simulink model "body_assembly"  (R2023b)
settings: Solver=VariableStepAuto  StartTime=0.0  StopTime=10.0  RelTol=1e-3
model workspace: external: MATLAB File S:\sabik\projects\3-1 project\3d modelling\body assembly 6\matlab_simulation\body_assembly_DataFile.m (data not in the file)
undefined symbols (not defined in the file or in its folder): smiData, X, Y, Z
libraries: sm_lib x393, nesl_utility x25, slpidlib x12
(part 8 of 8)

== system body_assembly/rocko_model/femur_fl/Assembly_SERVO_1_RIGID/Assembly_SERVO_stp_1_RIGID/Assembly_servo_inside_stp_1_RIGID ==
  ReferenceFrame : sm_lib/Frames and Transforms/Reference Frame
  Solid : sm_lib/Body Elements/File Solid  ExtGeomFileName=Assembly servo inside.stp_Default_sldprt.STEP  UnitType=FromFile  ExtGeomFileUnits=m  StepReaderType=HEX  ExportConvexHullGeometry=off  InertiaType=Custom  Mass=smiData.Solid(9).mass  MassUnits=kg  CenterOfMass=smiData.Solid(9).CoM  CenterOfMassUnits=mm  MomentsOfInertia=smiData.Solid(9).MoI  MomentsOfInertiaUnits=kg*mm^2  ProductsOfInertia=smiData.Solid(9).PoI  ProductsOfInertiaUnits=kg*mm^2  BasedOnType=DensityFromFile  Density=1000  DensityUnits=kg/m^3  DoExposeReferenceFrame=on  SerializedFrames=<Frames/>  GraphicType=FromGeometry  MarkerShape=Sphere  MarkerSize=10  GraphicVisPropType=SimpleVisualProperties  GraphicDiffuseColor=smiData.Solid(9).color  GraphicSpecularColor=[0.5 0.5 0.5 1.0]  GraphicAmbientColor=[0.15 0.15 0.15 1.0]  GraphicEmissiveColor=[0.0 0.0 0.0 1.0]  GraphicShininess=75  GraphicOpacity=smiData.Solid(9).opacity
  F : PMIOPort  Side=Left
  connections:
  Solid/RConn1 -- ReferenceFrame/RConn1 -- F/RConn1

== system body_assembly/rocko_model/femur_fl/Assembly_SERVO_1_RIGID/Assembly_SERVO_stp_1_RIGID/Assembly_servo_outside_stp_1_RIGID ==
  ReferenceFrame : sm_lib/Frames and Transforms/Reference Frame
  Solid : sm_lib/Body Elements/File Solid  ExtGeomFileName=Assembly servo outside.stp_Default_sldprt.STEP  UnitType=FromFile  ExtGeomFileUnits=m  StepReaderType=HEX  ExportConvexHullGeometry=off  InertiaType=Custom  Mass=smiData.Solid(8).mass  MassUnits=kg  CenterOfMass=smiData.Solid(8).CoM  CenterOfMassUnits=mm  MomentsOfInertia=smiData.Solid(8).MoI  MomentsOfInertiaUnits=kg*mm^2  ProductsOfInertia=smiData.Solid(8).PoI  ProductsOfInertiaUnits=kg*mm^2  BasedOnType=DensityFromFile  Density=1000  DensityUnits=kg/m^3  DoExposeReferenceFrame=on  SerializedFrames=<Frames/>  GraphicType=FromGeometry  MarkerShape=Sphere  MarkerSize=10  GraphicVisPropType=SimpleVisualProperties  GraphicDiffuseColor=smiData.Solid(8).color  GraphicSpecularColor=[0.5 0.5 0.5 1.0]  GraphicAmbientColor=[0.15 0.15 0.15 1.0]  GraphicEmissiveColor=[0.0 0.0 0.0 1.0]  GraphicShininess=75  GraphicOpacity=smiData.Solid(8).opacity
  F : PMIOPort  Side=Left
  connections:
  Solid/RConn1 -- ReferenceFrame/RConn1 -- F/RConn1

== system body_assembly/rocko_model/femur_fr/Assembly_SERVO_1_RIGID/Assembly_SERVO_stp_1_RIGID/Assembly_servo_inside_stp_1_RIGID ==
  ReferenceFrame : sm_lib/Frames and Transforms/Reference Frame
  Solid : sm_lib/Body Elements/File Solid  ExtGeomFileName=Assembly servo inside.stp_Default_sldprt.STEP  UnitType=FromFile  ExtGeomFileUnits=m  StepReaderType=HEX  ExportConvexHullGeometry=off  InertiaType=Custom  Mass=smiData.Solid(9).mass  MassUnits=kg  CenterOfMass=smiData.Solid(9).CoM  CenterOfMassUnits=mm  MomentsOfInertia=smiData.Solid(9).MoI  MomentsOfInertiaUnits=kg*mm^2  ProductsOfInertia=smiData.Solid(9).PoI  ProductsOfInertiaUnits=kg*mm^2  BasedOnType=DensityFromFile  Density=1000  DensityUnits=kg/m^3  DoExposeReferenceFrame=on  SerializedFrames=<Frames/>  GraphicType=FromGeometry  MarkerShape=Sphere  MarkerSize=10  GraphicVisPropType=SimpleVisualProperties  GraphicDiffuseColor=smiData.Solid(9).color  GraphicSpecularColor=[0.5 0.5 0.5 1.0]  GraphicAmbientColor=[0.15 0.15 0.15 1.0]  GraphicEmissiveColor=[0.0 0.0 0.0 1.0]  GraphicShininess=75  GraphicOpacity=smiData.Solid(9).opacity
  F : PMIOPort  Side=Left
  connections:
  Solid/RConn1 -- ReferenceFrame/RConn1 -- F/RConn1

== system body_assembly/rocko_model/femur_fr/Assembly_SERVO_1_RIGID/Assembly_SERVO_stp_1_RIGID/Assembly_servo_outside_stp_1_RIGID ==
  ReferenceFrame : sm_lib/Frames and Transforms/Reference Frame
  Solid : sm_lib/Body Elements/File Solid  ExtGeomFileName=Assembly servo outside.stp_Default_sldprt.STEP  UnitType=FromFile  ExtGeomFileUnits=m  StepReaderType=HEX  ExportConvexHullGeometry=off  InertiaType=Custom  Mass=smiData.Solid(8).mass  MassUnits=kg  CenterOfMass=smiData.Solid(8).CoM  CenterOfMassUnits=mm  MomentsOfInertia=smiData.Solid(8).MoI  MomentsOfInertiaUnits=kg*mm^2  ProductsOfInertia=smiData.Solid(8).PoI  ProductsOfInertiaUnits=kg*mm^2  BasedOnType=DensityFromFile  Density=1000  DensityUnits=kg/m^3  DoExposeReferenceFrame=on  SerializedFrames=<Frames/>  GraphicType=FromGeometry  MarkerShape=Sphere  MarkerSize=10  GraphicVisPropType=SimpleVisualProperties  GraphicDiffuseColor=smiData.Solid(8).color  GraphicSpecularColor=[0.5 0.5 0.5 1.0]  GraphicAmbientColor=[0.15 0.15 0.15 1.0]  GraphicEmissiveColor=[0.0 0.0 0.0 1.0]  GraphicShininess=75  GraphicOpacity=smiData.Solid(8).opacity
  F : PMIOPort  Side=Left
  connections:
  Solid/RConn1 -- ReferenceFrame/RConn1 -- F/RConn1

== matlab function body_assembly/back_left/MATLAB Function1 ==
  data: xd input; theta1d output; yd input; theta2d output; theta3d output; zd input
function [theta1d, theta2d, theta3d] = Inverse_Kinematics(xd, yd, zd)

len1 = 107;
len2 = 91;

theta3d = acos((xd^2 + yd^2 - len1^2 - len2^2) / (2*len1*len2));
theta1d = atan(yd/xd) - atan((len2 * sin(theta3d) / (len1 + len2*cos(theta3d))));


if(zd<=5)
    theta2d = -(pi/2)*sin((zd/5)*pi);
else
    theta2d = 0;
end

== matlab function body_assembly/front_right/MATLAB Function1 ==
  data: xd input; theta1d output; yd input; theta2d output; theta3d output; zd input
function [theta1d, theta2d, theta3d] = Inverse_Kinematics(xd, yd, zd)

len1 = 107;
len2 = 91;

theta3d = acos((xd^2 + yd^2 - len1^2 - len2^2) / (2*len1*len2));
theta1d = atan(yd/xd) - atan((len2 * sin(theta3d) / (len1 + len2*cos(theta3d))));


if(zd<=5)
    theta2d = -(pi/2)*sin((zd/5)*pi);
else
    theta2d = 0;
end

== matlab function body_assembly/back_left/MATLAB Function3 ==
  data: theta1 input; theta1d output; theta2 input; theta2d output; theta3d output; theta3 input
function [theta1d, theta2d, theta3d] = initial_angle_adjusted(theta1, theta2, theta3)

theta2d = theta2 + pi/2 ;
theta1d = theta1 - pi/4 + 10*pi/180;
theta3d = theta3 - 10*pi/180;

== matlab function body_assembly/back_left/desired_trajectory ==
  data: u input; xd output; yd output; zd output
function [xd, yd, zd] = Desired_Trajectory(u)

len1 = 107;
len2 = 91;

xd = 5;
yd = 130 - 50*sin(((u-7.63)/10)*2*pi) ;

zd = u;

== matlab function body_assembly/front_right/desired_trajectory ==
  data: u input; xd output; yd output; zd output
function [xd, yd, zd] = Desired_Trajectory(u)

len1 = 107;
len2 = 91;

xd = 5;
yd = 130 - 50*sin(((u-7.63)/10)*2*pi) ;

zd = u;

== matlab function body_assembly/back_right/MATLAB Function1 ==
  data: xd input; theta1d output; yd input; theta2d output; theta3d output; zd input
function [theta1d, theta2d, theta3d] = Inverse_Kinematics(xd, yd, zd)

len1 = 107;
len2 = 91;

theta3d = acos((xd^2 + yd^2 - len1^2 - len2^2) / (2*len1*len2));
theta1d = atan(yd/xd) - atan((len2 * sin(theta3d) / (len1 + len2*cos(theta3d))));


if(zd<=5)
    theta2d = -(pi/2)*sin((zd/5)*pi);
else
    theta2d = 0;
end

== matlab function body_assembly/front_right/MATLAB Function3 ==
  data: theta1 input; theta1d output; theta2 input; theta2d output; theta3d output; theta3 input
function [theta1d, theta2d, theta3d] = initial_angle_adjusted(theta1, theta2, theta3)

theta2d = theta2 + pi/2 ;
theta1d = theta1 - pi/4 + 10*pi/180;
theta3d = theta3 - 10*pi/180;

== matlab function body_assembly/back_right/MATLAB Function3 ==
  data: theta1 input; theta1d output; theta2 input; theta2d output; theta3d output; theta3 input
function [theta1d, theta2d, theta3d] = initial_angle_adjusted(theta1, theta2, theta3)

theta2d = theta2 + pi/2 ;
theta1d = theta1 - pi/4 + 10*pi/180;
theta3d = theta3 - 10*pi/180;

== matlab function body_assembly/back_right/desired_trajectory ==
  data: u input; xd output; yd output; zd output
function [xd, yd, zd] = Desired_Trajectory(u)

len1 = 107;
len2 = 91;

xd = 5;
yd = 130 - 50*sin(((u-7.63)/10)*2*pi) ;

zd = u;

== matlab function body_assembly/front_left/MATLAB Function1 ==
  data: xd input; theta1d output; yd input; theta2d output; theta3d output; zd input
function [theta1d, theta2d, theta3d] = Inverse_Kinematics(xd, yd, zd)

len1 = 107;
len2 = 91;

theta3d = acos((xd^2 + yd^2 - len1^2 - len2^2) / (2*len1*len2));
theta1d = atan(yd/xd) - atan((len2 * sin(theta3d) / (len1 + len2*cos(theta3d))));


if(zd<=5)
    theta2d = -(pi/2)*sin((zd/5)*pi);
else
    theta2d = 0;
end

== matlab function body_assembly/front_left/MATLAB Function3 ==
  data: theta1 input; theta1d output; theta2 input; theta2d output; theta3d output; theta3 input
function [theta1d, theta2d, theta3d] = initial_angle_adjusted(theta1, theta2, theta3)

theta2d = theta2 + pi/2 ;
theta1d = theta1 - pi/4 + 10*pi/180;
theta3d = theta3 - 10*pi/180;

== matlab function body_assembly/front_left/desired_trajectory ==
  data: u input; xd output; yd output; zd output
function [xd, yd, zd] = Desired_Trajectory(u)

len1 = 107;
len2 = 91;

xd = 5;
yd = 130 - 50*sin(((u-7.63)/10)*2*pi) ;

zd = u;
